simulink model "partial_delay_prog_test"  (Simulink 7.0)
settings: Solver=VariableStepDiscrete  StartTime=0.0  StopTime=500  RelTol=1e-3
libraries: xbsIndex_r4 x19, simulink x8
settings Model: Creator=User  LastModifiedBy=User
settings DebuggingCC: SaveWithDisabledLinksMsg=none  SaveWithParameterizedLinksMsg=none

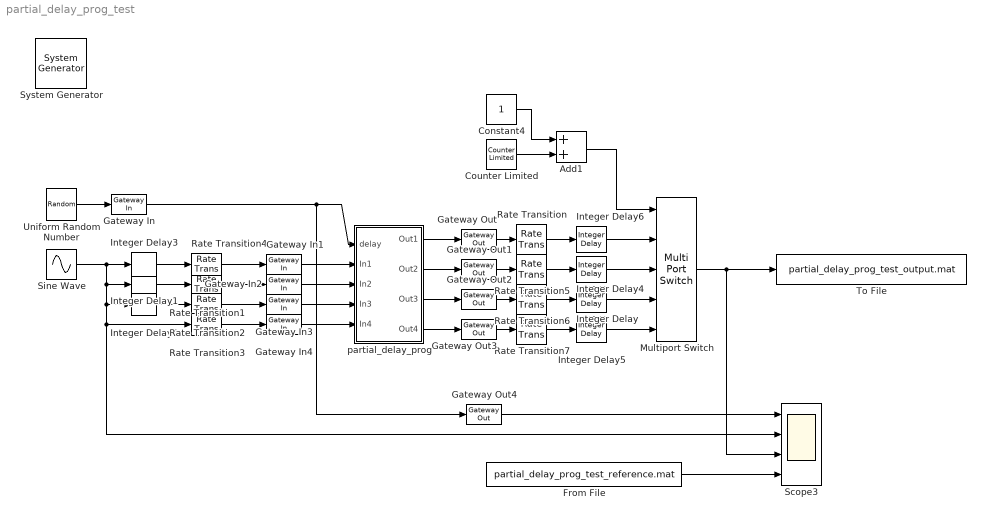
== system partial_delay_prog_test ==
  " System Generator" : xbsIndex_r4/ System Generator  Tag=genX  SystemSampleTime=-1  xilinxfamily=Virtex4  part=xc4vsx35  speed=-10  package=ff668  synthesis_tool=XST  clock_wrapper=Clock Enables  directory=./netlist  testbench=off  simulink_period=1  sysclk_period=100  dcm_input_clock_period=100  incr_netlist=off  trim_vbits=Everywhere in SubSystem  dbl_ovrd=According to Block Masks  core_generation=According to Block Masks  run_coregen=off  deprecated_control=off  eval_field=0  block_type=sysgen
      settings: block_version=10.1.1
  Add1 : Sum  OutDataType=sfix(16)  OutScaling=2^-10
  Constant4 : Constant  OutDataType=sfix(16)  OutScaling=2^0
  Counter Limited : simulink/Sources/Counter Limited  SystemSampleTime=-1  uplimit=3  tsamp=-1
  From File : FromFile  FileName=partial_delay_prog_test_reference.mat  SampleTime=0.25
  Gateway In : xbsIndex_r4/Gateway In  arith_type=Unsigned  n_bits=2  bin_pt=0  quantization=Truncate  overflow=Wrap  period=1  dbl_ovrd=off  timing_constraint=None  locs_specified=off  LOCs={}  block_type=gatewayin
      settings: infoedit="Gateway in block.  Converts inputs of type Simulink integer, double and fixed point to  Xilinx fixed point type.<P><P>Hardware notes:  In hardware these blocks become top level input ports."  block_version=10.1.1
  Gateway In{1..4} (4 alike) : xbsIndex_r4/Gateway In  arith_type="Signed  (2's comp)"  n_bits=8  bin_pt=7  quantization=Truncate  overflow=Wrap  period=1  dbl_ovrd=off  timing_constraint=None  locs_specified=off  LOCs={}  block_type=gatewayin
      settings: infoedit="Gateway in block.  Converts inputs of type Simulink integer, double and fixed point to  Xilinx fixed point type.<P><P>Hardware notes:  In hardware these blocks become top level input ports."  block_version=10.1.1
  Gateway Out{,1..4} (5 alike) : xbsIndex_r4/Gateway Out  hdl_port=on  timing_constraint=None  locs_specified=off  LOCs={}  block_type=gatewayout
      settings: infoedit="Gateway out block.  Converts Xilinx fixed point inputs into ouputs of type Simulink integer, double, or fixed point.<P><P>Hardware notes:  In hardware these blocks become top level output ports or are discarded, depending on how they are configured."  block_version=10.1.1
  Integer Delay : simulink/Discrete/Integer Delay  vinit=0.0  samptime=0.25  NumDelays=3
  Integer Delay1 : simulink/Discrete/Integer Delay  vinit=0.0  samptime=-1  NumDelays=2
  Integer Delay2 : simulink/Discrete/Integer Delay  vinit=0.0  samptime=-1  NumDelays=1
  Integer Delay3 : simulink/Discrete/Integer Delay  vinit=0.0  samptime=-1  NumDelays=3
  Integer Delay4 : simulink/Discrete/Integer Delay  vinit=0.0  samptime=0.25  NumDelays=2
  Integer Delay5 : simulink/Discrete/Integer Delay  vinit=0.0  samptime=0.25  NumDelays=4
  Integer Delay6 : simulink/Discrete/Integer Delay  vinit=0.0  samptime=0.25  NumDelays=1
  Multiport Switch : MultiPortSwitch  OutDataType=sfix(16)  OutScaling=2^0
  Rate Transition{,1..7} (8 alike) : RateTransition
  Scope3 : Scope  NumInputPorts=4
      settings: YMin=-5~-5~-5~-5  YMax=5~5~5~5
  Sine Wave : Sin  SineType=Sample based  SampleTime=0.25
  To File : ToFile  Filename=partial_delay_prog_test_output.mat  MatrixName=output
  Uniform Random Number : UniformRandomNumber  Minimum=0  Maximum=4  SampleTime=37
  partial_delay_prog : Subsystem  AncestorBlock=casper_library/Delays/partial_delay_prog  mask(partial_delay){n_inputs=4, mux_latency=2}
      mask prompts: n_inputs "Number of Inputs (? >= 2)"; mux_latency "Mux Latency"
      mask help:
      | For a set of parallel inputs which represent consecutive time samples of the
      | same input signal, this block delays the stream by a dynamically selectable
      | number of samples between 0 and (n_inputs-1).
      mask init:
      | partial_delay_init(gcb, ...
      |     'n_inputs', n_inputs, ...
      |     'mux_latency', mux_latency);
      mask Help: eval('xlWeb([getenv(''MLIB_ROOT''), ''\doc\htmlblocks\sp_partial_delay_prog\sp_partial_delay_prog.html''])')
  wires:
  Sine Wave/1 -> Integer Delay3/1, Integer Delay1/1, Integer Delay2/1, Rate Transition3/1, Scope3/2
  Uniform Random Number/1 -> Gateway In/1
  Gateway In/1 -> partial_delay_prog/1(delay), Gateway Out4/1
  Integer Delay3/1 -> Rate Transition4/1
  Integer Delay1/1 -> Rate Transition1/1
  Integer Delay2/1 -> Rate Transition2/1
  Gateway In1/1 -> partial_delay_prog/2(In1)
  Gateway In2/1 -> partial_delay_prog/3(In2)
  Gateway In3/1 -> partial_delay_prog/4(In3)
  Gateway In4/1 -> partial_delay_prog/5(In4)
  Rate Transition4/1 -> Gateway In1/1
  Rate Transition1/1 -> Gateway In2/1
  Rate Transition2/1 -> Gateway In3/1
  Rate Transition3/1 -> Gateway In4/1
  Constant4/1 -> Add1/1
  Counter Limited/1 -> Add1/2
  Add1/1 -> Multiport Switch/1
  partial_delay_prog/1(Out1) -> Gateway Out/1
  partial_delay_prog/2(Out2) -> Gateway Out1/1
  partial_delay_prog/3(Out3) -> Gateway Out2/1
  partial_delay_prog/4(Out4) -> Gateway Out3/1
  Gateway Out/1 -> Rate Transition/1
  Gateway Out1/1 -> Rate Transition5/1
  Gateway Out2/1 -> Rate Transition6/1
  Gateway Out3/1 -> Rate Transition7/1
  Rate Transition/1 -> Integer Delay6/1
  Rate Transition5/1 -> Integer Delay4/1
  Rate Transition6/1 -> Integer Delay/1
  Rate Transition7/1 -> Integer Delay5/1
  Integer Delay6/1 -> Multiport Switch/2
  Integer Delay4/1 -> Multiport Switch/3
  Integer Delay/1 -> Multiport Switch/4
  Integer Delay5/1 -> Multiport Switch/5
  Gateway Out4/1 -> Scope3/1
  Multiport Switch/1 -> Scope3/3, To File/1
  From File/1 -> Scope3/4

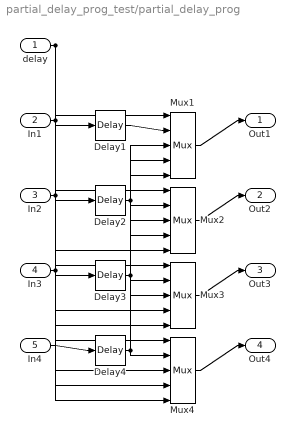
== system partial_delay_prog_test/partial_delay_prog ==
  delay : Inport  OutDataType=sfix(16)  OutScaling=2^0
  In1 : Inport  Port=2  OutDataType=sfix(16)  OutScaling=2^0
  In2 : Inport  Port=3  OutDataType=sfix(16)  OutScaling=2^0
  In3 : Inport  Port=4  OutDataType=sfix(16)  OutScaling=2^0
  In4 : Inport  Port=5  OutDataType=sfix(16)  OutScaling=2^0
  Delay{1..4} (4 alike) : xbsIndex_r4/Delay  en=off  latency=1  dbl_ovrd=off  reg_retiming=off  block_type=delay
      settings: xl_area=[0, 0, 0, 0, 0, 0, 0]  block_version=9.1.01
  Mux{1..4} (4 alike) : xbsIndex_r4/Mux  inputs=4  en=off  latency=2  precision=Full  arith_type="Signed  (2's comp)"  n_bits=8  bin_pt=2  quantization=Truncate  overflow=Wrap  dbl_ovrd=off  block_type=mux
      settings: xl_area=[0, 0, 0, 0, 0, 0, 0]  block_version=9.1.01
  Out1 : Outport  OutDataType=sfix(16)  OutScaling=2^0
  Out2 : Outport  Port=2  OutDataType=sfix(16)  OutScaling=2^0
  Out3 : Outport  Port=3  OutDataType=sfix(16)  OutScaling=2^0
  Out4 : Outport  Port=4  OutDataType=sfix(16)  OutScaling=2^0
  wires:
  In1/1 -> Delay1/1, Mux2/5, Mux3/4, Mux4/3
  Mux1/1 -> Out1/1
  delay/1 -> Mux1/1, Mux2/1, Mux3/1, Mux4/1
  Delay1/1 -> Mux1/2
  In2/1 -> Delay2/1, Mux3/5, Mux4/4
  Mux2/1 -> Out2/1
  Delay2/1 -> Mux2/2, Mux1/3
  In3/1 -> Delay3/1, Mux4/5
  Mux3/1 -> Out3/1
  Delay3/1 -> Mux3/2, Mux1/4, Mux2/3
  In4/1 -> Delay4/1
  Mux4/1 -> Out4/1
  Delay4/1 -> Mux4/2, Mux1/5, Mux2/4, Mux3/3
